simulink model "Wanchao_Shuttlecock_Parallel_with_Scaling"  (Simulink 7.7)
settings: Solver=ode4  StartTime=0.0  StopTime=inf  FixedStep=sample_time  RelTol=1e-3
InitFcn:
  | sample_time=0.005;%0.004;%0.0025;%0.02;
  | sample_time_Vicon = 0.005;
  | DeltaT = 0.02;
  | g = 9.81;
  | H0 = g%0.3165;
  | Kl = 1;
  | 
  | Omega_r = 1.6;%for Horizontal reference
  | Zeta_r = 0.7; %for Horizontal reference
  | Omega = 1.8;%for Horizontal Control
  | Zeta = 0.5;    %for Horizontal Control
  | 
  | Omega_h_r = 2.2; %for vertical reference
  | Zeta_h_r = 0.8;  %for vertical reference
  | Omega_h = 2.3;    %for vertical control
  | Zeta_h = 0.8;         %for vertical control
  | PI=pi;
  | 
  | Mass = 1;
  | Acc_Max = 4;
  | Acc_Max_h = 4;
  | 
  | Max_RP = 60;
  | 
  | % for NN
  | n = 5;
  | r = 3;
  | n2 = 5;
  | NN_ST = 0.02;
  | 
  | GAMA_V = 6;
  | gama_V_e = 0.01;
  | 
  | GAMA_W = GAMA_V;
  | gama_W_e =0.01;
  | 
  | % deadzone
  | NN_Deadzone_Z = 0;
  | 
  | % inputs nomalizaton parameters
  | NN_Z_y_min = -3;
  | NN_Z_y_max = 0.5;
  | 
  | NN_Z_v_max = 8;
  | NN_Z_v_min = -NN_Z_v_max;
  | 
  | % alpha = 0.034;
  | alpha = 1;
  | % c_f = 0.0015;
  | c_f = 0.001;
  | c_y_tilt = 1*0.5;
libraries: simulink x2, X330_Control x1
settings Model: Creator=ttcl3  LastModifiedBy=Vicon
settings SolverCC: MaxConsecutiveMinStep=auto
settings DebuggingCC: MultiTaskRateTransMsg=warning
settings SFSimCC: SimParseCustomCode=off

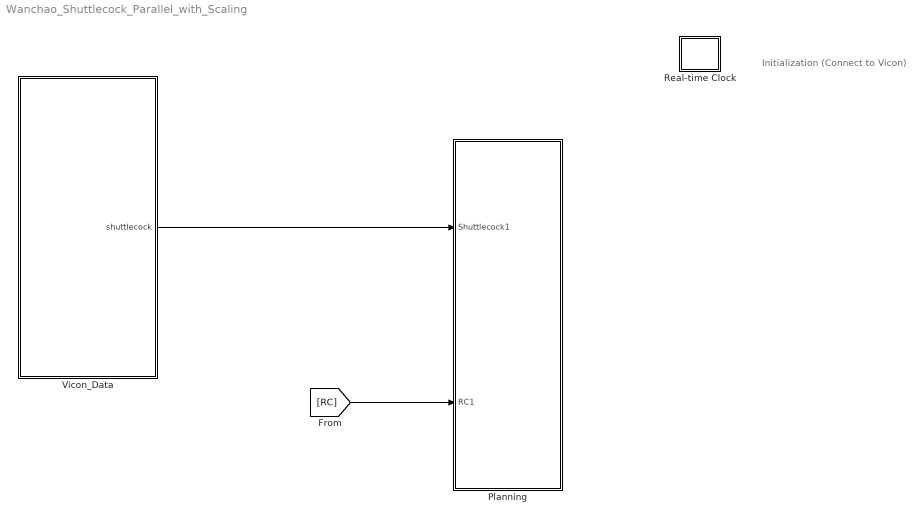
== system Wanchao_Shuttlecock_Parallel_with_Scaling ==
  note: Initialization
      | (Connect to Vicon)
  Planning : Subsystem
  Real-time Clock : Subsystem  mask(Real-time Clock){sample_time=0.02, tolerance=1}
      mask prompts: sample_time "Synchronize with real-time every n seconds:"; tolerance "Real-time warning tolerance (seconds):"
      mask help: Real-time Synchronization Block
      mask Help: This block synchronizes simulation time with the PC real-time clock or UNIX system clock. The first dialog entry is the period at which the clock is checked to insure real-time synchronization. The second dialog entry is the number of seconds that the simulation time must be within real-time before a warning is printed.
      mask Display: plot(0,0,100,100,[40,60,60,54,54,64,69,76,82,77,81,83,83,81,78,74,70,64,57,49,41,35,32,30,30,31,34,40,47,47,40,40],[90,90,85,85,80,79,76,87,80,70,64,57,49,41,33,28,24,22,21,23,25,31,37,46,56,65,73,78,80,85,85,90],[69,53,53],[64,50,73])
  Vicon_Data : Subsystem
  wires:
  Vicon_Data/1(shuttlecock) -> Planning/1(Shuttlecock1)
  [RC] -> Planning/2(RC1)

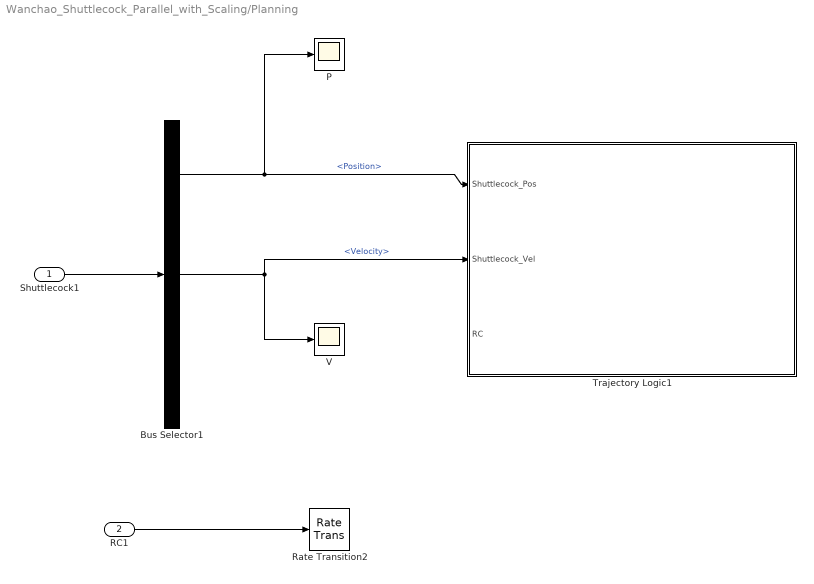
== system Wanchao_Shuttlecock_Parallel_with_Scaling/Planning ==
  Shuttlecock1 : Inport
  RC1 : Inport  Port=2
  Bus Selector1 : BusSelector  OutputSignals=Position,Velocity,Acceleration
  P : Scope
  Rate Transition2 : RateTransition  OutPortSampleTime=0.02
  Trajectory Logic1 : Subsystem
  V : Scope
  wires:
  RC1/1 -> Rate Transition2/1
  Shuttlecock1/1 -> Bus Selector1/1
  Bus Selector1/1 -> Trajectory Logic1/1(Shuttlecock_Pos), P/1  "<Position>"
  Bus Selector1/2 -> Trajectory Logic1/2(Shuttlecock_Vel), V/1  "<Velocity>"

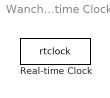
== system Wanchao_Shuttlecock_Parallel_with_Scaling/Real-time Clock ==
  Real-time Clock : S-Function  FunctionName=rtclock  Parameters=sample_time, tolerance  EnableBusSupport=off

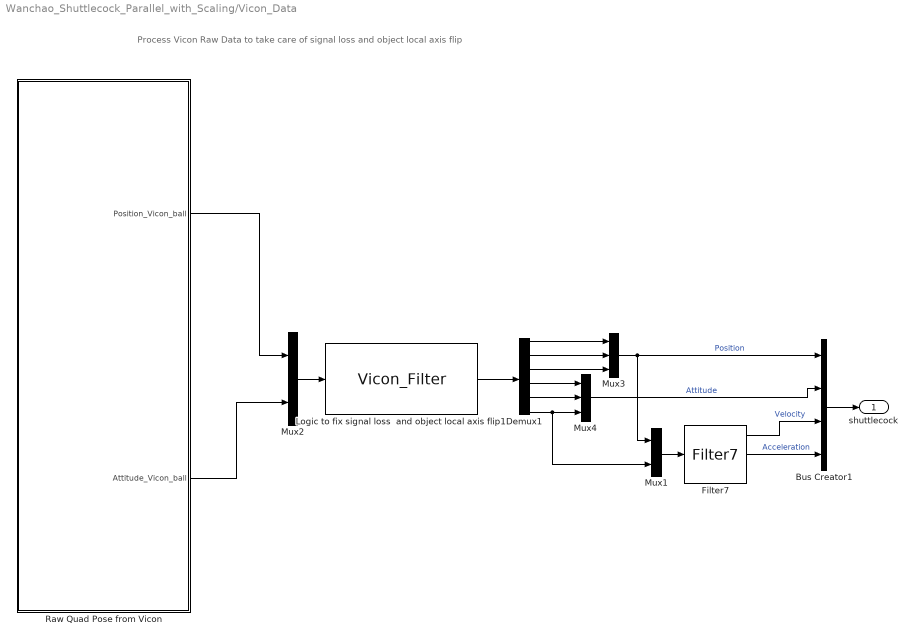
== system Wanchao_Shuttlecock_Parallel_with_Scaling/Vicon_Data ==
  note: Process Vicon Raw Data to take care of signal loss and object local axis flip
  Bus Creator1 : BusCreator
  Demux1 : Demux  Outputs=6
  Filter7 : X330_Control/Vicon Filter/Filter7  SystemSampleTime=-1
  Logic to fix signal loss  and object local axis flip1 : M-S-Function  FunctionName=Vicon_Filter
  Mux1 : Mux  Inputs=2
  Mux2 : Mux  Inputs=2
  Mux3 : Mux  Inputs=3
  Mux4 : Mux  Inputs=3
  Raw Quad Pose from Vicon : Subsystem
  shuttlecock : Outport
  wires:
  Mux2/1 -> Logic to fix signal loss  and object local axis flip1/1
  Logic to fix signal loss  and object local axis flip1/1 -> Demux1/1
  Demux1/3 -> Mux3/3
  Demux1/4 -> Mux4/1
  Demux1/5 -> Mux4/2
  Demux1/6 -> Mux4/3, Mux1/2
  Filter7/1 -> Bus Creator1/3  "Velocity"
  Filter7/2 -> Bus Creator1/4  "Acceleration"
  Mux4/1 -> Bus Creator1/2  "Attitude"
  Bus Creator1/1 -> shuttlecock/1
  Demux1/1 -> Mux3/1
  Demux1/2 -> Mux3/2
  Mux3/1 -> Mux1/1, Bus Creator1/1  "Position"
  Raw Quad Pose from Vicon/1(Position_Vicon_ball) -> Mux2/1
  Raw Quad Pose from Vicon/2(Attitude_Vicon_ball) -> Mux2/2
  Mux1/1 -> Filter7/1

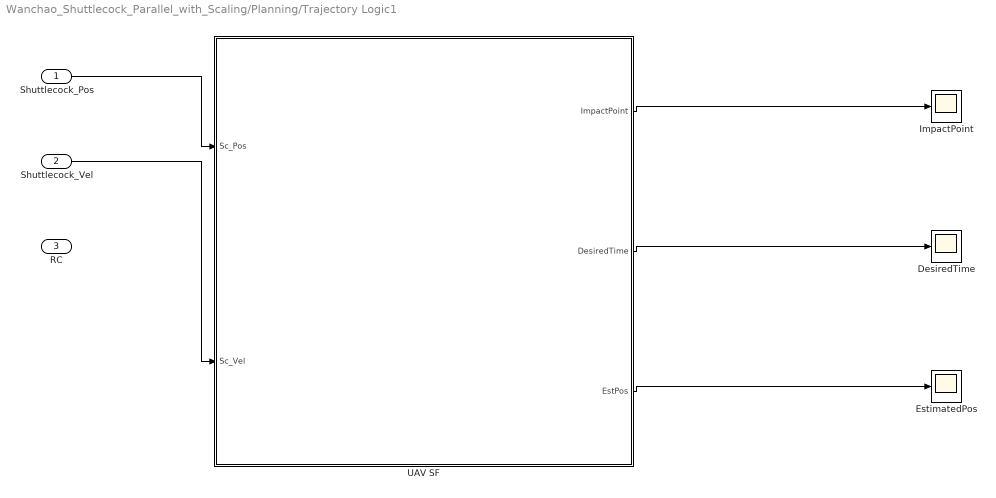
== system Wanchao_Shuttlecock_Parallel_with_Scaling/Planning/Trajectory Logic1 ==
  Shuttlecock_Pos : Inport
  Shuttlecock_Vel : Inport  Port=2
  RC : Inport  Port=3
  DesiredTime : Scope
      settings: SaveName=ScopeData3
  EstimatedPos : Scope
      settings: SaveName=ScopeData4
  ImpactPoint : Scope
      settings: SaveName=ScopeData2
  UAV SF : Stateflow chart  TreatAsAtomicUnit=on
  wires:
  Shuttlecock_Pos/1 -> UAV SF/1(Sc_Pos)
  Shuttlecock_Vel/1 -> UAV SF/2(Sc_Vel)
  UAV SF/1(ImpactPoint) -> ImpactPoint/1
  UAV SF/2(DesiredTime) -> DesiredTime/1
  UAV SF/3(EstPos) -> EstimatedPos/1

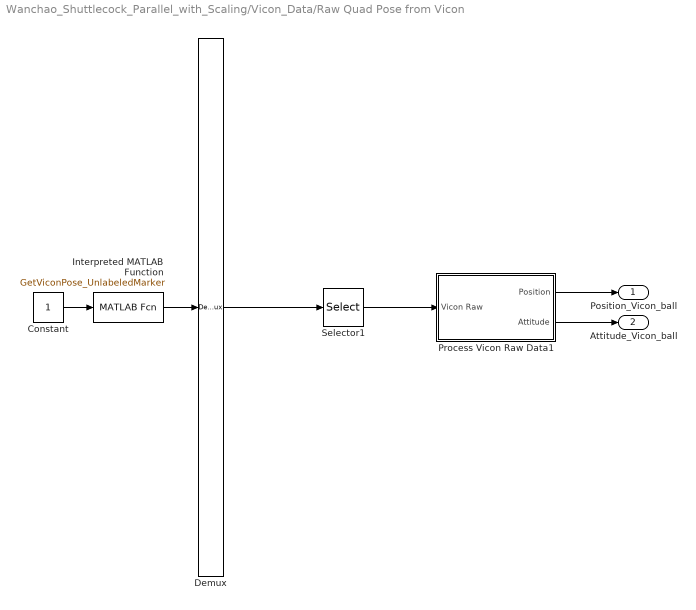
== system Wanchao_Shuttlecock_Parallel_with_Scaling/Vicon_Data/Raw Quad Pose from Vicon ==
  Constant : Constant
  Demux : Demux  Outputs=1
  Interpreted MATLAB Function : MATLABFcn  MATLABFcn=GetViconPose_UnlabeledMarker  OutputDimensions=30
  Process Vicon Raw Data1 : Subsystem
  Selector1 : Selector  InputPortWidth=30  IndexOptions=Index vector (dialog)  Indices=[1 2 3 ]  OutputSizes=1
  Position_Vicon_ball : Outport
  Attitude_Vicon_ball : Outport  Port=2
  wires:
  Interpreted MATLAB Function/1 -> Demux/1
  Constant/1 -> Interpreted MATLAB Function/1
  Process Vicon Raw Data1/2(Attitude) -> Attitude_Vicon_ball/1
  Process Vicon Raw Data1/1(Position) -> Position_Vicon_ball/1
  Selector1/1 -> Process Vicon Raw Data1/1(Vicon Raw)
  Demux/1 -> Selector1/1

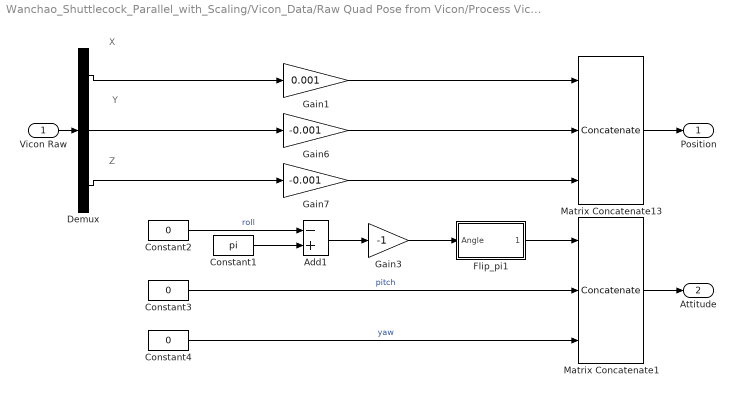
== system Wanchao_Shuttlecock_Parallel_with_Scaling/Vicon_Data/Raw Quad Pose from Vicon/Process Vicon Raw Data1 ==
  note: X
  note: Y
  note: Z
  Vicon Raw : Inport
  Add1 : Sum  Inputs=-+
  Constant1 : Constant  Value=pi  OutDataTypeStr=double
  Constant2 : Constant  Value=0  OutDataTypeStr=double
  Constant3 : Constant  Value=0  OutDataTypeStr=double
  Constant4 : Constant  Value=0  OutDataTypeStr=double
  Demux : Demux  Outputs=3
  Flip_pi1 : Subsystem
      mask Type: Flip -pi to pi
      mask Description: Flips the inputs into the range -pi to pi
      mask Help: Flips the inputs into the range -pi to pi
      mask Display: disp('Flip_pi')
  Gain1 : Gain  Gain=0.001
  Gain3 : Gain  Gain=-1
  Gain6 : Gain  Gain=-0.001
  Gain7 : Gain  Gain=-0.001
  Matrix Concatenate1 : Concatenate  NumInputs=3  Mode=Multidimensional array
  Matrix Concatenate13 : Concatenate  NumInputs=3  Mode=Multidimensional array
  Position : Outport
  Attitude : Outport  Port=2
  wires:
  Constant1/1 -> Add1/2
  Constant4/1 -> Matrix Concatenate1/3  "yaw"
  Gain1/1 -> Matrix Concatenate13/1
  Demux/1 -> Gain1/1
  Demux/2 -> Gain6/1
  Demux/3 -> Gain7/1
  Constant2/1 -> Add1/1  "roll"
  Gain6/1 -> Matrix Concatenate13/2
  Gain7/1 -> Matrix Concatenate13/3
  Add1/1 -> Gain3/1
  Gain3/1 -> Flip_pi1/1(Angle)
  Constant3/1 -> Matrix Concatenate1/2  "pitch"
  Flip_pi1/1(Angle_Flip) -> Matrix Concatenate1/1
  Matrix Concatenate13/1 -> Position/1
  Vicon Raw/1 -> Demux/1
  Matrix Concatenate1/1 -> Attitude/1

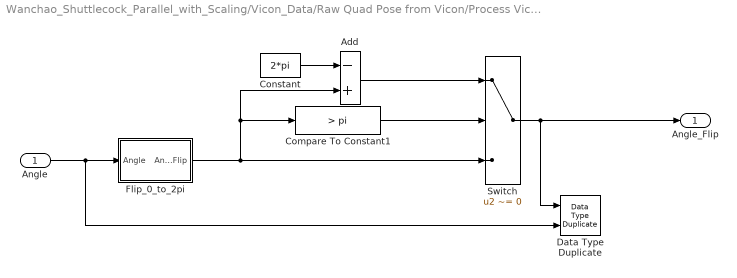
== system Wanchao_Shuttlecock_Parallel_with_Scaling/Vicon_Data/Raw Quad Pose from Vicon/Process Vicon Raw Data1/Flip_pi1 ==
  Angle : Inport
  Add : Sum  Inputs=-+
  Compare To Constant1 : simulink/Logic and Bit Operations/Compare To Constant  SystemSampleTime=-1  relop=>  const=pi  LogicOutDataTypeMode=uint8  ZeroCross=off
  Constant : Constant  Value=2*pi
  Data Type Duplicate : DataTypeDuplicate
  Flip_0_to_2pi : Subsystem
      mask Type: Flip zero to 2pi
      mask Description: Flips the inputs into the range zero to +2pi
      mask Help: Flips the inputs into the range zero to +2pi
      mask Display: disp('Flip_0_2pi')
  Switch : Switch  Criteria=u2 ~= 0
  Angle_Flip : Outport
  wires:
  Switch/1 -> Data Type Duplicate/1, Angle_Flip/1
  Add/1 -> Switch/1
  Constant/1 -> Add/1
  Compare To Constant1/1 -> Switch/2
  Flip_0_to_2pi/1(Angle_Flip) -> Add/2, Compare To Constant1/1, Switch/3
  Angle/1 -> Data Type Duplicate/2, Flip_0_to_2pi/1(Angle)

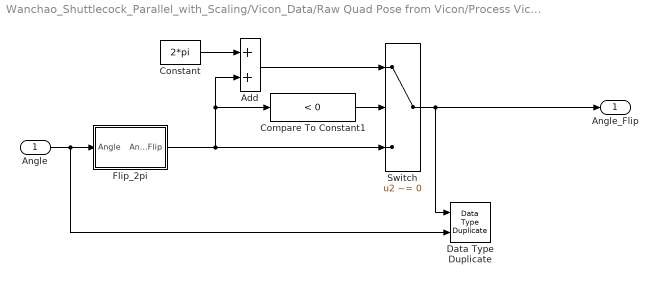
== system Wanchao_Shuttlecock_Parallel_with_Scaling/Vicon_Data/Raw Quad Pose from Vicon/Process Vicon Raw Data1/Flip_pi1/Flip_0_to_2pi ==
  Angle : Inport
  Add : Sum
  Compare To Constant1 : simulink/Logic and Bit Operations/Compare To Constant  SystemSampleTime=-1  relop=<  const=0  LogicOutDataTypeMode=uint8  ZeroCross=off
  Constant : Constant  Value=2*pi
  Data Type Duplicate : DataTypeDuplicate
  Flip_2pi : Subsystem
      mask Type: Flip -2pi to 2pi
      mask Description: Flips the inputs into the range -2pi to +2pi
      mask Help: Flips the inputs into the range -2pi to +2pi
      mask Display: disp('Flip_2pi')
  Switch : Switch  Criteria=u2 ~= 0
  Angle_Flip : Outport
  wires:
  Switch/1 -> Data Type Duplicate/1, Angle_Flip/1
  Angle/1 -> Data Type Duplicate/2, Flip_2pi/1(Angle)
  Add/1 -> Switch/1
  Constant/1 -> Add/1
  Compare To Constant1/1 -> Switch/2
  Flip_2pi/1(Angle_Flip) -> Switch/3, Add/2, Compare To Constant1/1

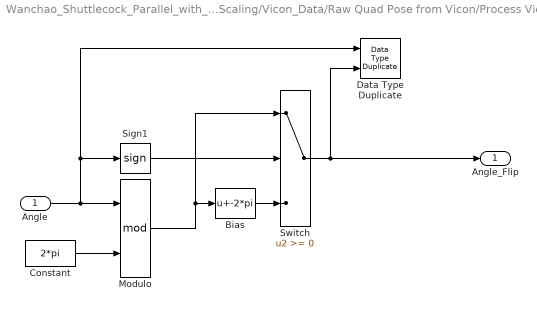
== system Wanchao_Shuttlecock_Parallel_with_Scaling/Vicon_Data/Raw Quad Pose from Vicon/Process Vicon Raw Data1/Flip_pi1/Flip_0_to_2pi/Flip_2pi ==
  Angle : Inport
  Bias : Bias  Bias=-2*pi
  Constant : Constant  Value=2*pi
  Data Type Duplicate : DataTypeDuplicate
  Modulo : Math  Operator=mod  SaturateOnIntegerOverflow=on
  Sign1 : Signum
  Switch : Switch
  Angle_Flip : Outport
  wires:
  Switch/1 -> Data Type Duplicate/2, Angle_Flip/1
  Bias/1 -> Switch/3
  Sign1/1 -> Switch/2
  Modulo/1 -> Switch/1, Bias/1
  Constant/1 -> Modulo/2
  Angle/1 -> Data Type Duplicate/1, Sign1/1, Modulo/1

== stateflow chart Planning/Trajectory Logic1/UAV SF ==
  state Airborne
    state Output1
      en:
      ImpactPoint[0] = X;
      ImpactPoint[1] = Y;
      ImpactPoint[2] = Z;
      DesiredTime = T;
    state TrajE
      en:
      E = Sc_Pos+Sc_Vel*DeltaT;
      [X,Y,Z,T] = Ball_Catching_Est(Sc_Pos[0],Sc_Pos[1],Sc_Pos[2],Sc_Vel[0],Sc_Vel[1],Sc_Vel[2],-0.5);
      EstPos = E;
    (default) -> (junction 7)
    (junction 7) -> (junction 13) [order 1] : [(abs(Sc_Pos[0]) <= 4.5)&(abs(Sc_Pos[1])<=4.5)&(abs(Sc_Pos[2])<=4)]
    TrajE -> Output1
    (junction 7) -> (junction 7) [order 2] : [(abs(Sc_Pos[0]) > 4.5)||(abs(Sc_Pos[1])>4.5)||(abs(Sc_Pos[2])>4)]
  (junction 12) -> (junction 8)
  (junction 11) -> (junction 12) [order 2]
  (junction 9) -> (junction 12)
  (junction 10) -> (junction 9) : {action1}
  (junction 11) -> (junction 10) [order 1] : [condition1]
  (default) -> (junction 11) : /* Check_Ball_Existence */
  data: xi function_input double; yi function_input double; zi function_input double; vxi function_input double; vyi function_input double; vzi function_input double; zd function_input double; x function_output double; y function_output double; z function_output double; time function_output double; ImpactPoint output double size=3; DesiredTime output double size=1; EstPos output uint8 size=3; Sc_Pos input double size=3; Sc_Vel input double size=3; DeltaT parameter double size=1; E local double size=3; V local double size=3; P local double size=3; T local double size=1; P1 local double size=3; T1 local double size=1; erP local double size=1; erT local double size=1; X local double; X1 local double; Y local double; Y1 local double; Z local double; Z1 local double
  function [x,y,z,time] = Ball_Catching_Est(xi,yi,zi,vxi,vyi,vzi,zd):
    | function [x,y,z,time] = Ball_Catching_Est(xi,yi,zi,vxi,vyi,vzi,zd)
    | 
    | g = 9.81;
    | m = 1;
    | 
    | t1 = (0-vzi)/g;
    | zmax = zi + vzi*t1 + 0.5*g*t1^2;
    | 
    | t2 = sqrt(2*(zd-zmax)/g);
    | time = t1+t2;
    | position = zeros(1,3);
    | x = xi + vxi*time;
    | y = yi + vyi*time;
    | z = zd;
